simulink model "control_PI_motor_DC"  (R2025b)
settings: Solver=ode45  StartTime=0.0  StopTime=5  RelTol=1e-3
settings Model: Creator=andre  LastModifiedBy=andre

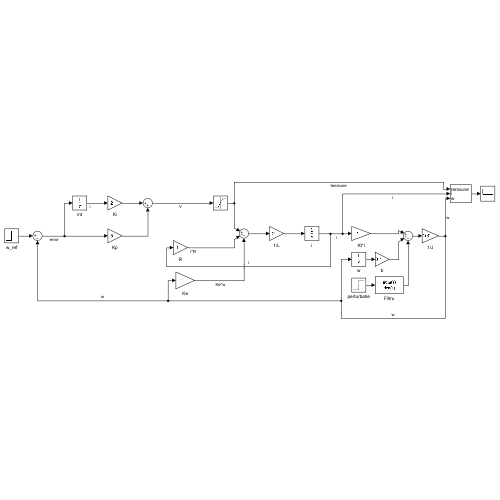
[thumbnail: Simulink's stored preview of the top-level diagram]
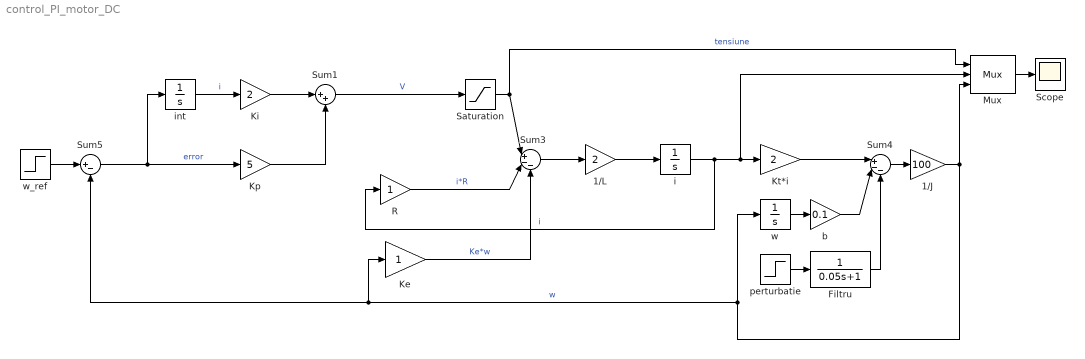
== system control_PI_motor_DC ==
  1/J : Gain  Gain=100
  1/L : Gain  Gain=2
  Filtru : TransferFcn  Denominator=[0.05 1]
  Ke : Gain
  Ki : Gain  Gain=2
  Kp : Gain  Gain=5
  Kt*i : Gain  Gain=2
  Mux : Mux  Inputs=3
      settings: DisplayOption=signals
  R : Gain
  Saturation : Saturate  UpperLimit=24  LowerLimit=-24
  Scope : Scope
      settings: ActiveDisplayYMinimum=-15.785817338683202  ActiveDisplayYMaximum=31.645542066236217
  Sum1 : Sum  Inputs=|++
  Sum3 : Sum  Inputs=|+--
  Sum4 : Sum  Inputs=|+--
  Sum5 : Sum  Inputs=|+-
  b : Gain  Gain=0.1
  i : Integrator
  int : Integrator
  perturbatie : Step  Time=2  After=3  SampleTime=0
  w : Integrator
  w_ref : Step  Time=0  After=10  SampleTime=0
  wires:
  int/1 -> Ki/1  "i"
  Ke/1 -> Sum3/3  "Ke*w"
  Sum4/1 -> 1/J/1
  w/1 -> b/1
  b/1 -> Sum4/2
  1/L/1 -> i/1
  i/1 -> Mux/2, Kt*i/1, R/1  "i"
  Kt*i/1 -> Sum4/1
  1/J/1 -> w/1, Sum5/2, Ke/1, Mux/3  "w"
  R/1 -> Sum3/2  "i*R"
  Sum5/1 -> int/1, Kp/1  "error"
  w_ref/1 -> Sum5/1
  Sum3/1 -> 1/L/1
  Kp/1 -> Sum1/2
  Ki/1 -> Sum1/1
  Sum1/1 -> Saturation/1  "V"
  Saturation/1 -> Mux/1, Sum3/1  "tensiune"
  perturbatie/1 -> Filtru/1
  Filtru/1 -> Sum4/3
  Mux/1 -> Scope/1
